simulink library "csu_grs_gravity_r_squared_lib"  (R2014b)
settings: Solver=ode45  StartTime=0.0  StopTime=10.0  RelTol=1e-3
undefined symbols (not defined in the file): central_body_gravity_mu
libraries: util_quat_lib x2, util_info_lib x1, util_common_lib x1
settings Model: Creator=mstewart  LastModifiedBy=mstewart

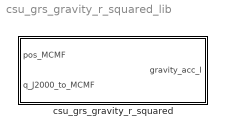
== system csu_grs_gravity_r_squared_lib ==
  csu_grs_gravity_r_squared : Subsystem  mask{mu_central_body=central_body_gravity_mu}
      mask prompts: mu_central_body "Mu paramater for central body"

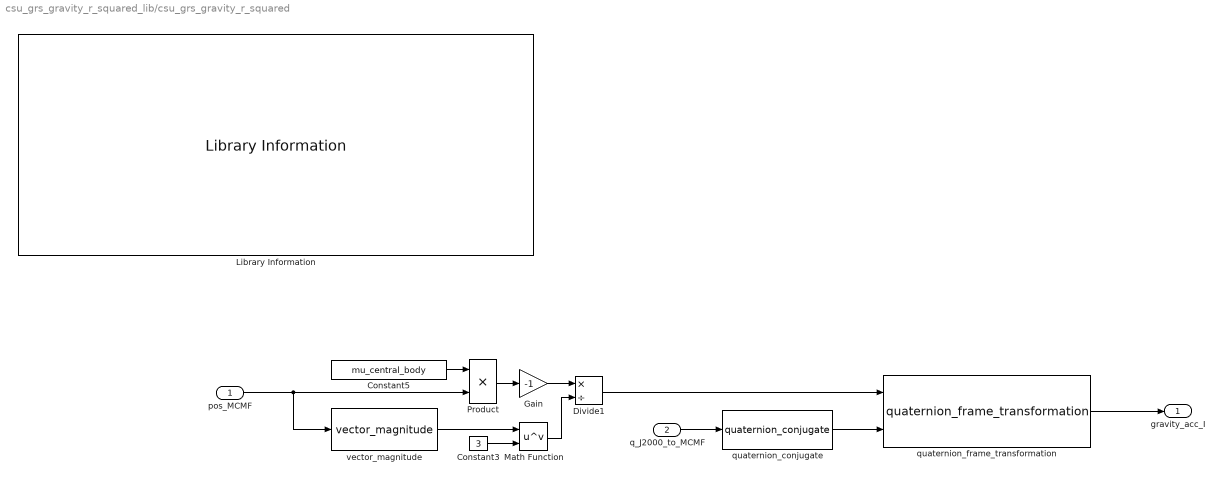
== system csu_grs_gravity_r_squared_lib/csu_grs_gravity_r_squared ==
  pos_MCMF : Inport
  q_J2000_to_MCMF : Inport  Port=2
  Constant3 : Constant  Value=3
  Constant5 : Constant  Value=mu_central_body
  Divide1 : Product  Inputs=*/
  Gain : Gain  Gain=-1
  Library Information : util_info_lib/Library Information  owner='NONE'
  Math Function : Math  Operator=pow  SaturateOnIntegerOverflow=on
  Product : Product  RndMeth=Zero
  quaternion_conjugate : util_quat_lib/quaternion_conjugate  SystemSampleTime=-1
  quaternion_frame_transformation : util_quat_lib/quaternion_frame_transformation  SystemSampleTime=-1
  vector_magnitude : util_common_lib/vector_magnitude  SystemSampleTime=-1
  gravity_acc_I : Outport
  wires:
  Divide1/1 -> quaternion_frame_transformation/1
  quaternion_conjugate/1 -> quaternion_frame_transformation/2
  quaternion_frame_transformation/1 -> gravity_acc_I/1
  q_J2000_to_MCMF/1 -> quaternion_conjugate/1
  Constant3/1 -> Math Function/2
  vector_magnitude/1 -> Math Function/1
  Gain/1 -> Divide1/1
  Product/1 -> Gain/1
  Constant5/1 -> Product/1
  pos_MCMF/1 -> Product/2, vector_magnitude/1
  Math Function/1 -> Divide1/2
